simulink model "power_microgrid_v5_battery"  (R2018b)
settings: Solver=ode23tb  StartTime=0.0  StopTime=24*60*60  FixedStep=1/(1000)  MaxStep=60  RelTol=1e-4
PreLoadFcn:
  | load('solar_load_data_24h.mat')
PostLoadFcn:
  | data = xlsread('Domestic_data_all_x3','Sheet1');
  | breakpoints1 = data(2:end,1)'
  | breakpoints2 = data(1,2:end)
  | table_data = data(2:end,2:end)
values from neighbouring files (symbols this model uses):
  SPD_1min = [0 0 0 0 0 0 0 0 0 0 0 0 ... (1441 elements, 1441x1)]    [default_PV_data.mat]
  SPT_1min = [0 60 120 180 240 300 360 420 480 540 600 660 ... (1441 elements, 1441x1)]    [default_PV_data.mat]
libraries: powerlib x155
(part 4 of 5)

== system power_microgrid_v5_battery/House 37 ==
  Clock : Clock
  Complex to Magnitude-Angle : ComplexToMagnitudeAngle  Output=Angle
  Controlled Current Source4 : powerlib/Electrical Sources/Controlled Current Source  Initialize=on  Source_Type=AC  Amplitude=0  Phase=0  Frequency=50  Measurements=None
      settings: SourceProductName=Simscape Electrical
  Gain10 : Gain  Gain=sqrt(2)
  Gain6 : Gain  Gain=-1/230
  Load Data 1-D Lookup Table : Lookup_n-D  NumberOfTableDimensions=1  BreakpointsForDimension1="[0.00\t600.00\t1200.00\t1800.00\t2400.00\t3000.00\t3600.00\t4200.00\t4800.00\t5400.00\t6000.00\t6600.00\t7200.00\t7800.00\t8400.00\t9000.00\t9600.00\t10200.00\t10800.00\t11400.00\t12000.00\t12600.00\t13200.00\t13800.00\t14400.00\t15000.00\t15600.00\t16200.00\t16800.00\t17400.00\t18000.00\t18600.00\t19200.00\t19800.00\t20400.00\t21000.00\t21600.00\t22200.00\t22800.00\t23400.00\t24000.00\t24600.00\t25200.00\t25800.00\t26400.00\t27000.00\t27600.00\t28200.00\t28800.00\t29400.00\t30000.00\t30600.00\t31200.00\t31800.00\t32400.00\t33000.00\t33600.00\t34200.00\t34800.00\t35400.00\t36000.00\t36600.00\t37200.00\t37800.00\t38400.00\t39000.00\t39600.00\t40200.00\t40800.00\t41400.00\t42000.00\t42600.00\t43200.00\t43800.00\t44400.00\t45000.00\t45600.00\t46200.00\t46800.00\t47400.00\t48000.00\t48600.00\t49200.00\t49800.00\t50400.00\t51000.00\t51600.00\t52200.00\t52800.00\t53400.00\t54000.00\t54600.00\t55200.00\t55800.00\t56400.00\t57000.00\t57600.00\t58200.00\t58800.00\t59400.00\t60000.00\t60600.00\t61200.00\t61800.00\t62400.00\t63000.00\t63600.00\t64200.00\t64800.00\t65400.00\t66000.00\t66600.00\t67200.00\t67800.00\t68400.00\t69000.00\t69600.00\t70200.00\t70800.00\t71400.00\t72000.00\t72600.00\t73200.00\t73800.00\t74400.00\t75000.00\t75600.00\t76200.00\t76800.00\t77400.00\t78000.00\t78600.00\t79200.00\t79800.00\t80400.00\t81000.00\t81600.00\t82200.00\t82800.00\t83400.00\t84000.00\t84600.00\t85200.00\t85800.00\t86400.00]"  BeginIndexSearchUsingPreviousIndexResult=on  Table="[287.9\t293.8\t263.0\t241.1\t234.1\t222.8\t214.5\t212.4\t211.1\t207.7\t200.9\t198.4\t194.4\t188.2\t185.8\t183.7\t189.6\t185.1\t179.0\t187.6\t179.7\t177.3\t169.0\t173.0\t169.3\t171.8\t165.9\t166.7\t170.5\t173.6\t179.5\t181.7\t196.2\t192.2\t177.7\t185.2\t250.8\t216.4\t218.6\t232.6\t256.0\t271.2\t292.1\t313.3\t326.6\t375.3\t421.6\t371.9\t375.5\t386.5\t395.4\t389.8\t364.4\t413.6\t395.4\t408.4\t410.4\t379.8\t364.2\t381.0\t383.4\t378.7\t384.3\t387.0\t365.1\t363.6\t369.7\t354.4\t367.8\t353.9\t361.0\t349.4\t377.3\t400.1\t383.7\t374.8\t382.5\t353.8\t359.6\t363.7\t347.9\t331.7\t346.5\t345.9\t334.7\t324.2\t332.7\t349.6\t363.2\t345.4\t350.9\t355.6\t374.0\t393.2\t389.1\t383.8\t404.1\t426.3\t443.7\t449.0\t452.4\t452.9\t477.6\t496.2\t496.4\t518.8\t529.6\t538.5\t545.1\t587.6\t591.8\t593.3\t586.6\t595.1\t603.6\t621.9\t603.6\t607.2\t582.9\t601.9\t605.1\t579.6\t566.2\t557.6\t554.0\t551.3\t552.4\t585.1\t576.4\t564.1\t559.0\t553.1\t536.3\t517.7\t521.5\t519.5\t485.4\t437.7\t418.5\t395.9\t370.8\t353.7\t336.4\t311.0\t287.9]"  InternalRulePriority=Speed  RndMeth=Simplest  InputSameDT=on
  Magnitude-Angle to Complex1 : MagnitudeAngleToComplex
  Snubber3 : powerlib/Elements/Series RLC Branch  LConnTagsString=__new0  RConnTagsString=__new0  BranchType=R  Resistance=1e6  Inductance=1e-3  SetiL0=off  InitialCurrent=0  Capacitance=1e-6  Setx0=off  InitialVoltage=0  Measurements=None
      settings: SourceProductName=Simscape Electrical
  meas cur2 : powerlib/Measurements/Current Measurement  PhasorSimulation=on  OutputType=Complex  PSBequivalent=0
      settings: SourceProductName=Simscape Electrical
  Conn1 : PMIOPort  Side=Left
  Conn2 : PMIOPort  Port=2  Side=Right
  Out1 : Outport
  wires:
  meas cur2/1 -> Out1/1
  Clock/1 -> Load Data 1-D Lookup Table/1
  Magnitude-Angle to Complex1/1 -> Controlled Current Source4/1
  Load Data 1-D Lookup Table/1 -> Gain6/1
  Complex to Magnitude-Angle/1 -> Magnitude-Angle to Complex1/2
  Gain10/1 -> Magnitude-Angle to Complex1/1
  Gain6/1 -> Gain10/1
  [Vsec] -> Complex to Magnitude-Angle/1
  connections:
  Conn1/RConn1 -- meas cur2/LConn1
  Snubber3/LConn1 -- meas cur2/RConn1 -- Controlled Current Source4/RConn1
  Snubber3/RConn1 -- Controlled Current Source4/LConn1 -- Conn2/RConn1

== system power_microgrid_v5_battery/House 38 ==
  Clock : Clock
  Complex to Magnitude-Angle : ComplexToMagnitudeAngle  Output=Angle
  Controlled Current Source4 : powerlib/Electrical Sources/Controlled Current Source  Initialize=on  Source_Type=AC  Amplitude=0  Phase=0  Frequency=50  Measurements=None
      settings: SourceProductName=Simscape Electrical
  Gain10 : Gain  Gain=sqrt(2)
  Gain6 : Gain  Gain=-1/230
  Load Data 1-D Lookup Table : Lookup_n-D  NumberOfTableDimensions=1  BreakpointsForDimension1="[0.00\t600.00\t1200.00\t1800.00\t2400.00\t3000.00\t3600.00\t4200.00\t4800.00\t5400.00\t6000.00\t6600.00\t7200.00\t7800.00\t8400.00\t9000.00\t9600.00\t10200.00\t10800.00\t11400.00\t12000.00\t12600.00\t13200.00\t13800.00\t14400.00\t15000.00\t15600.00\t16200.00\t16800.00\t17400.00\t18000.00\t18600.00\t19200.00\t19800.00\t20400.00\t21000.00\t21600.00\t22200.00\t22800.00\t23400.00\t24000.00\t24600.00\t25200.00\t25800.00\t26400.00\t27000.00\t27600.00\t28200.00\t28800.00\t29400.00\t30000.00\t30600.00\t31200.00\t31800.00\t32400.00\t33000.00\t33600.00\t34200.00\t34800.00\t35400.00\t36000.00\t36600.00\t37200.00\t37800.00\t38400.00\t39000.00\t39600.00\t40200.00\t40800.00\t41400.00\t42000.00\t42600.00\t43200.00\t43800.00\t44400.00\t45000.00\t45600.00\t46200.00\t46800.00\t47400.00\t48000.00\t48600.00\t49200.00\t49800.00\t50400.00\t51000.00\t51600.00\t52200.00\t52800.00\t53400.00\t54000.00\t54600.00\t55200.00\t55800.00\t56400.00\t57000.00\t57600.00\t58200.00\t58800.00\t59400.00\t60000.00\t60600.00\t61200.00\t61800.00\t62400.00\t63000.00\t63600.00\t64200.00\t64800.00\t65400.00\t66000.00\t66600.00\t67200.00\t67800.00\t68400.00\t69000.00\t69600.00\t70200.00\t70800.00\t71400.00\t72000.00\t72600.00\t73200.00\t73800.00\t74400.00\t75000.00\t75600.00\t76200.00\t76800.00\t77400.00\t78000.00\t78600.00\t79200.00\t79800.00\t80400.00\t81000.00\t81600.00\t82200.00\t82800.00\t83400.00\t84000.00\t84600.00\t85200.00\t85800.00\t86400.00]"  BeginIndexSearchUsingPreviousIndexResult=on  Table="[287.9\t293.8\t263.0\t241.1\t234.1\t222.8\t214.5\t212.4\t211.1\t207.7\t200.9\t198.4\t194.4\t188.2\t185.8\t183.7\t189.6\t185.1\t179.0\t187.6\t179.7\t177.3\t169.0\t173.0\t169.3\t171.8\t165.9\t166.7\t170.5\t173.6\t179.5\t181.7\t196.2\t192.2\t177.7\t185.2\t250.8\t216.4\t218.6\t232.6\t256.0\t271.2\t292.1\t313.3\t326.6\t375.3\t421.6\t371.9\t375.5\t386.5\t395.4\t389.8\t364.4\t413.6\t395.4\t408.4\t410.4\t379.8\t364.2\t381.0\t383.4\t378.7\t384.3\t387.0\t365.1\t363.6\t369.7\t354.4\t367.8\t353.9\t361.0\t349.4\t377.3\t400.1\t383.7\t374.8\t382.5\t353.8\t359.6\t363.7\t347.9\t331.7\t346.5\t345.9\t334.7\t324.2\t332.7\t349.6\t363.2\t345.4\t350.9\t355.6\t374.0\t393.2\t389.1\t383.8\t404.1\t426.3\t443.7\t449.0\t452.4\t452.9\t477.6\t496.2\t496.4\t518.8\t529.6\t538.5\t545.1\t587.6\t591.8\t593.3\t586.6\t595.1\t603.6\t621.9\t603.6\t607.2\t582.9\t601.9\t605.1\t579.6\t566.2\t557.6\t554.0\t551.3\t552.4\t585.1\t576.4\t564.1\t559.0\t553.1\t536.3\t517.7\t521.5\t519.5\t485.4\t437.7\t418.5\t395.9\t370.8\t353.7\t336.4\t311.0\t287.9]"  InternalRulePriority=Speed  RndMeth=Simplest  InputSameDT=on
  Magnitude-Angle to Complex1 : MagnitudeAngleToComplex
  Snubber3 : powerlib/Elements/Series RLC Branch  LConnTagsString=__new0  RConnTagsString=__new0  BranchType=R  Resistance=1e6  Inductance=1e-3  SetiL0=off  InitialCurrent=0  Capacitance=1e-6  Setx0=off  InitialVoltage=0  Measurements=None
      settings: SourceProductName=Simscape Electrical
  meas cur2 : powerlib/Measurements/Current Measurement  PhasorSimulation=on  OutputType=Complex  PSBequivalent=0
      settings: SourceProductName=Simscape Electrical
  Conn1 : PMIOPort  Side=Left
  Conn2 : PMIOPort  Port=2  Side=Right
  Out1 : Outport
  wires:
  meas cur2/1 -> Out1/1
  Clock/1 -> Load Data 1-D Lookup Table/1
  Magnitude-Angle to Complex1/1 -> Controlled Current Source4/1
  Load Data 1-D Lookup Table/1 -> Gain6/1
  Complex to Magnitude-Angle/1 -> Magnitude-Angle to Complex1/2
  Gain10/1 -> Magnitude-Angle to Complex1/1
  Gain6/1 -> Gain10/1
  [Vsec] -> Complex to Magnitude-Angle/1
  connections:
  Conn1/RConn1 -- meas cur2/LConn1
  Snubber3/LConn1 -- meas cur2/RConn1 -- Controlled Current Source4/RConn1
  Snubber3/RConn1 -- Controlled Current Source4/LConn1 -- Conn2/RConn1

== system power_microgrid_v5_battery/House 39 ==
  Clock : Clock
  Complex to Magnitude-Angle : ComplexToMagnitudeAngle  Output=Angle
  Controlled Current Source4 : powerlib/Electrical Sources/Controlled Current Source  Initialize=on  Source_Type=AC  Amplitude=0  Phase=0  Frequency=50  Measurements=None
      settings: SourceProductName=Simscape Electrical
  Gain10 : Gain  Gain=sqrt(2)
  Gain6 : Gain  Gain=-1/230
  Load Data 1-D Lookup Table : Lookup_n-D  NumberOfTableDimensions=1  BreakpointsForDimension1="[0.00\t600.00\t1200.00\t1800.00\t2400.00\t3000.00\t3600.00\t4200.00\t4800.00\t5400.00\t6000.00\t6600.00\t7200.00\t7800.00\t8400.00\t9000.00\t9600.00\t10200.00\t10800.00\t11400.00\t12000.00\t12600.00\t13200.00\t13800.00\t14400.00\t15000.00\t15600.00\t16200.00\t16800.00\t17400.00\t18000.00\t18600.00\t19200.00\t19800.00\t20400.00\t21000.00\t21600.00\t22200.00\t22800.00\t23400.00\t24000.00\t24600.00\t25200.00\t25800.00\t26400.00\t27000.00\t27600.00\t28200.00\t28800.00\t29400.00\t30000.00\t30600.00\t31200.00\t31800.00\t32400.00\t33000.00\t33600.00\t34200.00\t34800.00\t35400.00\t36000.00\t36600.00\t37200.00\t37800.00\t38400.00\t39000.00\t39600.00\t40200.00\t40800.00\t41400.00\t42000.00\t42600.00\t43200.00\t43800.00\t44400.00\t45000.00\t45600.00\t46200.00\t46800.00\t47400.00\t48000.00\t48600.00\t49200.00\t49800.00\t50400.00\t51000.00\t51600.00\t52200.00\t52800.00\t53400.00\t54000.00\t54600.00\t55200.00\t55800.00\t56400.00\t57000.00\t57600.00\t58200.00\t58800.00\t59400.00\t60000.00\t60600.00\t61200.00\t61800.00\t62400.00\t63000.00\t63600.00\t64200.00\t64800.00\t65400.00\t66000.00\t66600.00\t67200.00\t67800.00\t68400.00\t69000.00\t69600.00\t70200.00\t70800.00\t71400.00\t72000.00\t72600.00\t73200.00\t73800.00\t74400.00\t75000.00\t75600.00\t76200.00\t76800.00\t77400.00\t78000.00\t78600.00\t79200.00\t79800.00\t80400.00\t81000.00\t81600.00\t82200.00\t82800.00\t83400.00\t84000.00\t84600.00\t85200.00\t85800.00\t86400.00]"  BeginIndexSearchUsingPreviousIndexResult=on  Table="[239.5\t239.3\t230.7\t221.1\t236.7\t224.0\t212.7\t208.1\t198.4\t189.5\t188.5\t190.5\t188.9\t175.4\t181.1\t172.1\t176.3\t181.6\t168.9\t165.2\t160.0\t171.7\t173.3\t158.7\t161.2\t183.5\t182.5\t185.8\t174.7\t172.1\t172.3\t171.8\t196.0\t196.8\t185.5\t191.4\t195.5\t211.1\t225.6\t240.9\t294.0\t327.5\t322.1\t404.9\t489.6\t440.2\t382.2\t398.2\t392.8\t423.0\t511.9\t472.7\t420.5\t405.4\t368.1\t353.8\t392.6\t414.0\t406.8\t409.2\t418.6\t483.6\t444.8\t421.6\t429.0\t444.4\t466.1\t457.6\t477.5\t422.1\t438.5\t445.5\t481.4\t506.4\t471.7\t425.1\t441.5\t411.9\t413.0\t436.9\t429.4\t446.6\t455.6\t465.0\t461.5\t475.0\t453.6\t447.1\t473.5\t480.7\t494.8\t468.2\t491.4\t470.2\t471.6\t525.4\t540.8\t554.3\t565.1\t626.5\t743.4\t744.6\t717.5\t733.8\t778.9\t822.7\t807.8\t820.4\t832.5\t863.5\t825.7\t764.6\t774.5\t717.8\t709.4\t778.0\t738.5\t753.7\t739.0\t770.0\t756.2\t812.2\t746.3\t716.1\t705.9\t737.2\t679.1\t623.3\t583.2\t563.0\t523.2\t504.6\t460.7\t440.9\t392.2\t372.0\t362.3\t339.5\t315.3\t289.8\t274.7\t275.1\t266.0\t264.5\t239.5]"  InternalRulePriority=Speed  RndMeth=Simplest  InputSameDT=on
  Magnitude-Angle to Complex1 : MagnitudeAngleToComplex
  Snubber3 : powerlib/Elements/Series RLC Branch  LConnTagsString=__new0  RConnTagsString=__new0  BranchType=R  Resistance=1e6  Inductance=1e-3  SetiL0=off  InitialCurrent=0  Capacitance=1e-6  Setx0=off  InitialVoltage=0  Measurements=None
      settings: SourceProductName=Simscape Electrical
  meas cur2 : powerlib/Measurements/Current Measurement  PhasorSimulation=on  OutputType=Complex  PSBequivalent=0
      settings: SourceProductName=Simscape Electrical
  Conn1 : PMIOPort  Side=Left
  Conn2 : PMIOPort  Port=2  Side=Right
  Out1 : Outport
  wires:
  Magnitude-Angle to Complex1/1 -> Controlled Current Source4/1
  meas cur2/1 -> Out1/1
  Clock/1 -> Load Data 1-D Lookup Table/1
  Load Data 1-D Lookup Table/1 -> Gain6/1
  [Vsec] -> Complex to Magnitude-Angle/1
  Gain6/1 -> Gain10/1
  Gain10/1 -> Magnitude-Angle to Complex1/1
  Complex to Magnitude-Angle/1 -> Magnitude-Angle to Complex1/2
  connections:
  meas cur2/LConn1 -- Conn1/RConn1
  Snubber3/LConn1 -- Controlled Current Source4/RConn1 -- meas cur2/RConn1
  Snubber3/RConn1 -- Controlled Current Source4/LConn1 -- Conn2/RConn1

== system power_microgrid_v5_battery/House 4 ==
  Clock : Clock
  Complex to Magnitude-Angle : ComplexToMagnitudeAngle  Output=Angle
  Controlled Current Source4 : powerlib/Electrical Sources/Controlled Current Source  Initialize=on  Source_Type=AC  Amplitude=0  Phase=0  Frequency=50  Measurements=None
      settings: SourceProductName=Simscape Electrical
  Gain10 : Gain  Gain=sqrt(2)
  Gain6 : Gain  Gain=-1/230
  Load Data 1-D Lookup Table : Lookup_n-D  NumberOfTableDimensions=1  BreakpointsForDimension1="[0.00\t600.00\t1200.00\t1800.00\t2400.00\t3000.00\t3600.00\t4200.00\t4800.00\t5400.00\t6000.00\t6600.00\t7200.00\t7800.00\t8400.00\t9000.00\t9600.00\t10200.00\t10800.00\t11400.00\t12000.00\t12600.00\t13200.00\t13800.00\t14400.00\t15000.00\t15600.00\t16200.00\t16800.00\t17400.00\t18000.00\t18600.00\t19200.00\t19800.00\t20400.00\t21000.00\t21600.00\t22200.00\t22800.00\t23400.00\t24000.00\t24600.00\t25200.00\t25800.00\t26400.00\t27000.00\t27600.00\t28200.00\t28800.00\t29400.00\t30000.00\t30600.00\t31200.00\t31800.00\t32400.00\t33000.00\t33600.00\t34200.00\t34800.00\t35400.00\t36000.00\t36600.00\t37200.00\t37800.00\t38400.00\t39000.00\t39600.00\t40200.00\t40800.00\t41400.00\t42000.00\t42600.00\t43200.00\t43800.00\t44400.00\t45000.00\t45600.00\t46200.00\t46800.00\t47400.00\t48000.00\t48600.00\t49200.00\t49800.00\t50400.00\t51000.00\t51600.00\t52200.00\t52800.00\t53400.00\t54000.00\t54600.00\t55200.00\t55800.00\t56400.00\t57000.00\t57600.00\t58200.00\t58800.00\t59400.00\t60000.00\t60600.00\t61200.00\t61800.00\t62400.00\t63000.00\t63600.00\t64200.00\t64800.00\t65400.00\t66000.00\t66600.00\t67200.00\t67800.00\t68400.00\t69000.00\t69600.00\t70200.00\t70800.00\t71400.00\t72000.00\t72600.00\t73200.00\t73800.00\t74400.00\t75000.00\t75600.00\t76200.00\t76800.00\t77400.00\t78000.00\t78600.00\t79200.00\t79800.00\t80400.00\t81000.00\t81600.00\t82200.00\t82800.00\t83400.00\t84000.00\t84600.00\t85200.00\t85800.00\t86400.00]"  BeginIndexSearchUsingPreviousIndexResult=on  Table="[179.5\t163.3\t152.9\t132.5\t118.9\t111.3\t124.6\t103.3\t83.5\t81.2\t85.9\t85.2\t91.9\t95.6\t95.9\t81.8\t83.7\t86.7\t93.8\t81.2\t92.7\t99.4\t112.6\t88.2\t85.6\t78.4\t88.4\t93.9\t86.1\t86.0\t111.7\t143.5\t122.7\t136.8\t142.2\t135.1\t145.6\t141.8\t152.1\t140.3\t167.9\t256.6\t226.1\t263.8\t283.9\t303.3\t279.5\t294.9\t282.3\t288.8\t333.5\t360.9\t421.4\t494.2\t392.5\t439.7\t395.9\t394.4\t364.9\t353.0\t359.1\t370.9\t398.5\t447.4\t344.5\t330.8\t306.8\t331.3\t331.9\t307.6\t371.3\t387.4\t376.6\t360.2\t414.1\t445.1\t411.1\t389.5\t425.2\t340.0\t316.3\t332.8\t352.3\t301.8\t261.8\t298.1\t350.9\t327.8\t296.5\t319.6\t368.4\t327.2\t265.7\t277.9\t292.9\t301.4\t377.9\t336.0\t324.6\t353.8\t389.7\t355.9\t328.4\t325.9\t378.1\t338.0\t379.1\t414.8\t418.1\t464.8\t488.1\t489.1\t485.7\t581.3\t579.7\t526.2\t551.4\t618.6\t628.5\t578.8\t553.3\t481.5\t455.6\t487.9\t507.3\t497.6\t515.4\t510.2\t490.5\t500.5\t494.1\t532.9\t506.5\t466.6\t438.0\t385.4\t381.2\t385.9\t351.7\t371.3\t340.8\t320.2\t277.0\t228.9\t179.5]"  InternalRulePriority=Speed  RndMeth=Simplest  InputSameDT=on
  Magnitude-Angle to Complex1 : MagnitudeAngleToComplex
  Snubber3 : powerlib/Elements/Series RLC Branch  LConnTagsString=__new0  RConnTagsString=__new0  BranchType=R  Resistance=1e6  Inductance=1e-3  SetiL0=off  InitialCurrent=0  Capacitance=1e-6  Setx0=off  InitialVoltage=0  Measurements=None
      settings: SourceProductName=Simscape Electrical
  meas cur2 : powerlib/Measurements/Current Measurement  PhasorSimulation=on  OutputType=Complex  PSBequivalent=0
      settings: SourceProductName=Simscape Electrical
  Conn1 : PMIOPort  Side=Left
  Conn2 : PMIOPort  Port=2  Side=Right
  Out1 : Outport
  wires:
  meas cur2/1 -> Out1/1
  Clock/1 -> Load Data 1-D Lookup Table/1
  Magnitude-Angle to Complex1/1 -> Controlled Current Source4/1
  Load Data 1-D Lookup Table/1 -> Gain6/1
  Complex to Magnitude-Angle/1 -> Magnitude-Angle to Complex1/2
  Gain10/1 -> Magnitude-Angle to Complex1/1
  Gain6/1 -> Gain10/1
  [Vsec] -> Complex to Magnitude-Angle/1
  connections:
  Conn1/RConn1 -- meas cur2/LConn1
  Snubber3/LConn1 -- meas cur2/RConn1 -- Controlled Current Source4/RConn1
  Snubber3/RConn1 -- Controlled Current Source4/LConn1 -- Conn2/RConn1

== system power_microgrid_v5_battery/House 40 ==
  Clock : Clock
  Complex to Magnitude-Angle : ComplexToMagnitudeAngle  Output=Angle
  Controlled Current Source4 : powerlib/Electrical Sources/Controlled Current Source  Initialize=on  Source_Type=AC  Amplitude=0  Phase=0  Frequency=50  Measurements=None
      settings: SourceProductName=Simscape Electrical
  Gain10 : Gain  Gain=sqrt(2)
  Gain6 : Gain  Gain=-1/230
  Load Data 1-D Lookup Table : Lookup_n-D  NumberOfTableDimensions=1  BreakpointsForDimension1="[0.00\t600.00\t1200.00\t1800.00\t2400.00\t3000.00\t3600.00\t4200.00\t4800.00\t5400.00\t6000.00\t6600.00\t7200.00\t7800.00\t8400.00\t9000.00\t9600.00\t10200.00\t10800.00\t11400.00\t12000.00\t12600.00\t13200.00\t13800.00\t14400.00\t15000.00\t15600.00\t16200.00\t16800.00\t17400.00\t18000.00\t18600.00\t19200.00\t19800.00\t20400.00\t21000.00\t21600.00\t22200.00\t22800.00\t23400.00\t24000.00\t24600.00\t25200.00\t25800.00\t26400.00\t27000.00\t27600.00\t28200.00\t28800.00\t29400.00\t30000.00\t30600.00\t31200.00\t31800.00\t32400.00\t33000.00\t33600.00\t34200.00\t34800.00\t35400.00\t36000.00\t36600.00\t37200.00\t37800.00\t38400.00\t39000.00\t39600.00\t40200.00\t40800.00\t41400.00\t42000.00\t42600.00\t43200.00\t43800.00\t44400.00\t45000.00\t45600.00\t46200.00\t46800.00\t47400.00\t48000.00\t48600.00\t49200.00\t49800.00\t50400.00\t51000.00\t51600.00\t52200.00\t52800.00\t53400.00\t54000.00\t54600.00\t55200.00\t55800.00\t56400.00\t57000.00\t57600.00\t58200.00\t58800.00\t59400.00\t60000.00\t60600.00\t61200.00\t61800.00\t62400.00\t63000.00\t63600.00\t64200.00\t64800.00\t65400.00\t66000.00\t66600.00\t67200.00\t67800.00\t68400.00\t69000.00\t69600.00\t70200.00\t70800.00\t71400.00\t72000.00\t72600.00\t73200.00\t73800.00\t74400.00\t75000.00\t75600.00\t76200.00\t76800.00\t77400.00\t78000.00\t78600.00\t79200.00\t79800.00\t80400.00\t81000.00\t81600.00\t82200.00\t82800.00\t83400.00\t84000.00\t84600.00\t85200.00\t85800.00\t86400.00]"  BeginIndexSearchUsingPreviousIndexResult=on  Table="[239.5\t239.3\t230.7\t221.1\t236.7\t224.0\t212.7\t208.1\t198.4\t189.5\t188.5\t190.5\t188.9\t175.4\t181.1\t172.1\t176.3\t181.6\t168.9\t165.2\t160.0\t171.7\t173.3\t158.7\t161.2\t183.5\t182.5\t185.8\t174.7\t172.1\t172.3\t171.8\t196.0\t196.8\t185.5\t191.4\t195.5\t211.1\t225.6\t240.9\t294.0\t327.5\t322.1\t404.9\t489.6\t440.2\t382.2\t398.2\t392.8\t423.0\t511.9\t472.7\t420.5\t405.4\t368.1\t353.8\t392.6\t414.0\t406.8\t409.2\t418.6\t483.6\t444.8\t421.6\t429.0\t444.4\t466.1\t457.6\t477.5\t422.1\t438.5\t445.5\t481.4\t506.4\t471.7\t425.1\t441.5\t411.9\t413.0\t436.9\t429.4\t446.6\t455.6\t465.0\t461.5\t475.0\t453.6\t447.1\t473.5\t480.7\t494.8\t468.2\t491.4\t470.2\t471.6\t525.4\t540.8\t554.3\t565.1\t626.5\t743.4\t744.6\t717.5\t733.8\t778.9\t822.7\t807.8\t820.4\t832.5\t863.5\t825.7\t764.6\t774.5\t717.8\t709.4\t778.0\t738.5\t753.7\t739.0\t770.0\t756.2\t812.2\t746.3\t716.1\t705.9\t737.2\t679.1\t623.3\t583.2\t563.0\t523.2\t504.6\t460.7\t440.9\t392.2\t372.0\t362.3\t339.5\t315.3\t289.8\t274.7\t275.1\t266.0\t264.5\t239.5]"  InternalRulePriority=Speed  RndMeth=Simplest  InputSameDT=on
  Magnitude-Angle to Complex1 : MagnitudeAngleToComplex
  Snubber3 : powerlib/Elements/Series RLC Branch  LConnTagsString=__new0  RConnTagsString=__new0  BranchType=R  Resistance=1e6  Inductance=1e-3  SetiL0=off  InitialCurrent=0  Capacitance=1e-6  Setx0=off  InitialVoltage=0  Measurements=None
      settings: SourceProductName=Simscape Electrical
  meas cur2 : powerlib/Measurements/Current Measurement  PhasorSimulation=on  OutputType=Complex  PSBequivalent=0
      settings: SourceProductName=Simscape Electrical
  Conn1 : PMIOPort  Side=Left
  Conn2 : PMIOPort  Port=2  Side=Right
  Out1 : Outport
  wires:
  meas cur2/1 -> Out1/1
  Clock/1 -> Load Data 1-D Lookup Table/1
  Magnitude-Angle to Complex1/1 -> Controlled Current Source4/1
  Load Data 1-D Lookup Table/1 -> Gain6/1
  Complex to Magnitude-Angle/1 -> Magnitude-Angle to Complex1/2
  Gain10/1 -> Magnitude-Angle to Complex1/1
  Gain6/1 -> Gain10/1
  [Vsec] -> Complex to Magnitude-Angle/1
  connections:
  Controlled Current Source4/LConn1 -- Conn2/RConn1 -- Snubber3/RConn1
  Controlled Current Source4/RConn1 -- meas cur2/RConn1 -- Snubber3/LConn1
  Conn1/RConn1 -- meas cur2/LConn1

== system power_microgrid_v5_battery/House 41 ==
  Clock : Clock
  Complex to Magnitude-Angle : ComplexToMagnitudeAngle  Output=Angle
  Controlled Current Source4 : powerlib/Electrical Sources/Controlled Current Source  Initialize=on  Source_Type=AC  Amplitude=0  Phase=0  Frequency=50  Measurements=None
      settings: SourceProductName=Simscape Electrical
  Gain10 : Gain  Gain=sqrt(2)
  Gain6 : Gain  Gain=-1/230
  Load Data 1-D Lookup Table : Lookup_n-D  NumberOfTableDimensions=1  BreakpointsForDimension1="[0.00\t600.00\t1200.00\t1800.00\t2400.00\t3000.00\t3600.00\t4200.00\t4800.00\t5400.00\t6000.00\t6600.00\t7200.00\t7800.00\t8400.00\t9000.00\t9600.00\t10200.00\t10800.00\t11400.00\t12000.00\t12600.00\t13200.00\t13800.00\t14400.00\t15000.00\t15600.00\t16200.00\t16800.00\t17400.00\t18000.00\t18600.00\t19200.00\t19800.00\t20400.00\t21000.00\t21600.00\t22200.00\t22800.00\t23400.00\t24000.00\t24600.00\t25200.00\t25800.00\t26400.00\t27000.00\t27600.00\t28200.00\t28800.00\t29400.00\t30000.00\t30600.00\t31200.00\t31800.00\t32400.00\t33000.00\t33600.00\t34200.00\t34800.00\t35400.00\t36000.00\t36600.00\t37200.00\t37800.00\t38400.00\t39000.00\t39600.00\t40200.00\t40800.00\t41400.00\t42000.00\t42600.00\t43200.00\t43800.00\t44400.00\t45000.00\t45600.00\t46200.00\t46800.00\t47400.00\t48000.00\t48600.00\t49200.00\t49800.00\t50400.00\t51000.00\t51600.00\t52200.00\t52800.00\t53400.00\t54000.00\t54600.00\t55200.00\t55800.00\t56400.00\t57000.00\t57600.00\t58200.00\t58800.00\t59400.00\t60000.00\t60600.00\t61200.00\t61800.00\t62400.00\t63000.00\t63600.00\t64200.00\t64800.00\t65400.00\t66000.00\t66600.00\t67200.00\t67800.00\t68400.00\t69000.00\t69600.00\t70200.00\t70800.00\t71400.00\t72000.00\t72600.00\t73200.00\t73800.00\t74400.00\t75000.00\t75600.00\t76200.00\t76800.00\t77400.00\t78000.00\t78600.00\t79200.00\t79800.00\t80400.00\t81000.00\t81600.00\t82200.00\t82800.00\t83400.00\t84000.00\t84600.00\t85200.00\t85800.00\t86400.00]"  BeginIndexSearchUsingPreviousIndexResult=on  Table="[179.5\t163.3\t152.9\t132.5\t118.9\t111.3\t124.6\t103.3\t83.5\t81.2\t85.9\t85.2\t91.9\t95.6\t95.9\t81.8\t83.7\t86.7\t93.8\t81.2\t92.7\t99.4\t112.6\t88.2\t85.6\t78.4\t88.4\t93.9\t86.1\t86.0\t111.7\t143.5\t122.7\t136.8\t142.2\t135.1\t145.6\t141.8\t152.1\t140.3\t167.9\t256.6\t226.1\t263.8\t283.9\t303.3\t279.5\t294.9\t282.3\t288.8\t333.5\t360.9\t421.4\t494.2\t392.5\t439.7\t395.9\t394.4\t364.9\t353.0\t359.1\t370.9\t398.5\t447.4\t344.5\t330.8\t306.8\t331.3\t331.9\t307.6\t371.3\t387.4\t376.6\t360.2\t414.1\t445.1\t411.1\t389.5\t425.2\t340.0\t316.3\t332.8\t352.3\t301.8\t261.8\t298.1\t350.9\t327.8\t296.5\t319.6\t368.4\t327.2\t265.7\t277.9\t292.9\t301.4\t377.9\t336.0\t324.6\t353.8\t389.7\t355.9\t328.4\t325.9\t378.1\t338.0\t379.1\t414.8\t418.1\t464.8\t488.1\t489.1\t485.7\t581.3\t579.7\t526.2\t551.4\t618.6\t628.5\t578.8\t553.3\t481.5\t455.6\t487.9\t507.3\t497.6\t515.4\t510.2\t490.5\t500.5\t494.1\t532.9\t506.5\t466.6\t438.0\t385.4\t381.2\t385.9\t351.7\t371.3\t340.8\t320.2\t277.0\t228.9\t179.5]"  InternalRulePriority=Speed  RndMeth=Simplest  InputSameDT=on
  Magnitude-Angle to Complex1 : MagnitudeAngleToComplex
  Snubber3 : powerlib/Elements/Series RLC Branch  LConnTagsString=__new0  RConnTagsString=__new0  BranchType=R  Resistance=1e6  Inductance=1e-3  SetiL0=off  InitialCurrent=0  Capacitance=1e-6  Setx0=off  InitialVoltage=0  Measurements=None
      settings: SourceProductName=Simscape Electrical
  meas cur2 : powerlib/Measurements/Current Measurement  PhasorSimulation=on  OutputType=Complex  PSBequivalent=0
      settings: SourceProductName=Simscape Electrical
  Conn1 : PMIOPort  Side=Left
  Conn2 : PMIOPort  Port=2  Side=Right
  Out1 : Outport
  wires:
  meas cur2/1 -> Out1/1
  Clock/1 -> Load Data 1-D Lookup Table/1
  Magnitude-Angle to Complex1/1 -> Controlled Current Source4/1
  Load Data 1-D Lookup Table/1 -> Gain6/1
  Complex to Magnitude-Angle/1 -> Magnitude-Angle to Complex1/2
  Gain10/1 -> Magnitude-Angle to Complex1/1
  Gain6/1 -> Gain10/1
  [Vsec] -> Complex to Magnitude-Angle/1
  connections:
  Conn1/RConn1 -- meas cur2/LConn1
  Snubber3/LConn1 -- meas cur2/RConn1 -- Controlled Current Source4/RConn1
  Snubber3/RConn1 -- Controlled Current Source4/LConn1 -- Conn2/RConn1

== system power_microgrid_v5_battery/House 5 ==
  Clock : Clock
  Complex to Magnitude-Angle : ComplexToMagnitudeAngle  Output=Angle
  Controlled Current Source4 : powerlib/Electrical Sources/Controlled Current Source  Initialize=on  Source_Type=AC  Amplitude=0  Phase=0  Frequency=50  Measurements=None
      settings: SourceProductName=Simscape Electrical
  Gain10 : Gain  Gain=sqrt(2)
  Gain6 : Gain  Gain=-1/230
  Load Data 1-D Lookup Table : Lookup_n-D  NumberOfTableDimensions=1  BreakpointsForDimension1="[0.00\t600.00\t1200.00\t1800.00\t2400.00\t3000.00\t3600.00\t4200.00\t4800.00\t5400.00\t6000.00\t6600.00\t7200.00\t7800.00\t8400.00\t9000.00\t9600.00\t10200.00\t10800.00\t11400.00\t12000.00\t12600.00\t13200.00\t13800.00\t14400.00\t15000.00\t15600.00\t16200.00\t16800.00\t17400.00\t18000.00\t18600.00\t19200.00\t19800.00\t20400.00\t21000.00\t21600.00\t22200.00\t22800.00\t23400.00\t24000.00\t24600.00\t25200.00\t25800.00\t26400.00\t27000.00\t27600.00\t28200.00\t28800.00\t29400.00\t30000.00\t30600.00\t31200.00\t31800.00\t32400.00\t33000.00\t33600.00\t34200.00\t34800.00\t35400.00\t36000.00\t36600.00\t37200.00\t37800.00\t38400.00\t39000.00\t39600.00\t40200.00\t40800.00\t41400.00\t42000.00\t42600.00\t43200.00\t43800.00\t44400.00\t45000.00\t45600.00\t46200.00\t46800.00\t47400.00\t48000.00\t48600.00\t49200.00\t49800.00\t50400.00\t51000.00\t51600.00\t52200.00\t52800.00\t53400.00\t54000.00\t54600.00\t55200.00\t55800.00\t56400.00\t57000.00\t57600.00\t58200.00\t58800.00\t59400.00\t60000.00\t60600.00\t61200.00\t61800.00\t62400.00\t63000.00\t63600.00\t64200.00\t64800.00\t65400.00\t66000.00\t66600.00\t67200.00\t67800.00\t68400.00\t69000.00\t69600.00\t70200.00\t70800.00\t71400.00\t72000.00\t72600.00\t73200.00\t73800.00\t74400.00\t75000.00\t75600.00\t76200.00\t76800.00\t77400.00\t78000.00\t78600.00\t79200.00\t79800.00\t80400.00\t81000.00\t81600.00\t82200.00\t82800.00\t83400.00\t84000.00\t84600.00\t85200.00\t85800.00\t86400.00]"  BeginIndexSearchUsingPreviousIndexResult=on  Table="[179.5\t163.3\t152.9\t132.5\t118.9\t111.3\t124.6\t103.3\t83.5\t81.2\t85.9\t85.2\t91.9\t95.6\t95.9\t81.8\t83.7\t86.7\t93.8\t81.2\t92.7\t99.4\t112.6\t88.2\t85.6\t78.4\t88.4\t93.9\t86.1\t86.0\t111.7\t143.5\t122.7\t136.8\t142.2\t135.1\t145.6\t141.8\t152.1\t140.3\t167.9\t256.6\t226.1\t263.8\t283.9\t303.3\t279.5\t294.9\t282.3\t288.8\t333.5\t360.9\t421.4\t494.2\t392.5\t439.7\t395.9\t394.4\t364.9\t353.0\t359.1\t370.9\t398.5\t447.4\t344.5\t330.8\t306.8\t331.3\t331.9\t307.6\t371.3\t387.4\t376.6\t360.2\t414.1\t445.1\t411.1\t389.5\t425.2\t340.0\t316.3\t332.8\t352.3\t301.8\t261.8\t298.1\t350.9\t327.8\t296.5\t319.6\t368.4\t327.2\t265.7\t277.9\t292.9\t301.4\t377.9\t336.0\t324.6\t353.8\t389.7\t355.9\t328.4\t325.9\t378.1\t338.0\t379.1\t414.8\t418.1\t464.8\t488.1\t489.1\t485.7\t581.3\t579.7\t526.2\t551.4\t618.6\t628.5\t578.8\t553.3\t481.5\t455.6\t487.9\t507.3\t497.6\t515.4\t510.2\t490.5\t500.5\t494.1\t532.9\t506.5\t466.6\t438.0\t385.4\t381.2\t385.9\t351.7\t371.3\t340.8\t320.2\t277.0\t228.9\t179.5]"  InternalRulePriority=Speed  RndMeth=Simplest  InputSameDT=on
  Magnitude-Angle to Complex1 : MagnitudeAngleToComplex
  Snubber3 : powerlib/Elements/Series RLC Branch  LConnTagsString=__new0  RConnTagsString=__new0  BranchType=R  Resistance=1e6  Inductance=1e-3  SetiL0=off  InitialCurrent=0  Capacitance=1e-6  Setx0=off  InitialVoltage=0  Measurements=None
      settings: SourceProductName=Simscape Electrical
  meas cur2 : powerlib/Measurements/Current Measurement  PhasorSimulation=on  OutputType=Complex  PSBequivalent=0
      settings: SourceProductName=Simscape Electrical
  Conn1 : PMIOPort  Side=Left
  Conn2 : PMIOPort  Port=2  Side=Right
  Out1 : Outport
  wires:
  meas cur2/1 -> Out1/1
  Clock/1 -> Load Data 1-D Lookup Table/1
  Magnitude-Angle to Complex1/1 -> Controlled Current Source4/1
  Load Data 1-D Lookup Table/1 -> Gain6/1
  Complex to Magnitude-Angle/1 -> Magnitude-Angle to Complex1/2
  Gain10/1 -> Magnitude-Angle to Complex1/1
  Gain6/1 -> Gain10/1
  [Vsec] -> Complex to Magnitude-Angle/1
  connections:
  Conn1/RConn1 -- meas cur2/LConn1
  Snubber3/LConn1 -- meas cur2/RConn1 -- Controlled Current Source4/RConn1
  Snubber3/RConn1 -- Controlled Current Source4/LConn1 -- Conn2/RConn1

== system power_microgrid_v5_battery/House 6 ==
  Clock : Clock
  Complex to Magnitude-Angle : ComplexToMagnitudeAngle  Output=Angle
  Controlled Current Source4 : powerlib/Electrical Sources/Controlled Current Source  Initialize=on  Source_Type=AC  Amplitude=0  Phase=0  Frequency=50  Measurements=None
      settings: SourceProductName=Simscape Electrical
  Gain10 : Gain  Gain=sqrt(2)
  Gain6 : Gain  Gain=-1/230
  Load Data 1-D Lookup Table : Lookup_n-D  NumberOfTableDimensions=1  BreakpointsForDimension1="[0.00\t600.00\t1200.00\t1800.00\t2400.00\t3000.00\t3600.00\t4200.00\t4800.00\t5400.00\t6000.00\t6600.00\t7200.00\t7800.00\t8400.00\t9000.00\t9600.00\t10200.00\t10800.00\t11400.00\t12000.00\t12600.00\t13200.00\t13800.00\t14400.00\t15000.00\t15600.00\t16200.00\t16800.00\t17400.00\t18000.00\t18600.00\t19200.00\t19800.00\t20400.00\t21000.00\t21600.00\t22200.00\t22800.00\t23400.00\t24000.00\t24600.00\t25200.00\t25800.00\t26400.00\t27000.00\t27600.00\t28200.00\t28800.00\t29400.00\t30000.00\t30600.00\t31200.00\t31800.00\t32400.00\t33000.00\t33600.00\t34200.00\t34800.00\t35400.00\t36000.00\t36600.00\t37200.00\t37800.00\t38400.00\t39000.00\t39600.00\t40200.00\t40800.00\t41400.00\t42000.00\t42600.00\t43200.00\t43800.00\t44400.00\t45000.00\t45600.00\t46200.00\t46800.00\t47400.00\t48000.00\t48600.00\t49200.00\t49800.00\t50400.00\t51000.00\t51600.00\t52200.00\t52800.00\t53400.00\t54000.00\t54600.00\t55200.00\t55800.00\t56400.00\t57000.00\t57600.00\t58200.00\t58800.00\t59400.00\t60000.00\t60600.00\t61200.00\t61800.00\t62400.00\t63000.00\t63600.00\t64200.00\t64800.00\t65400.00\t66000.00\t66600.00\t67200.00\t67800.00\t68400.00\t69000.00\t69600.00\t70200.00\t70800.00\t71400.00\t72000.00\t72600.00\t73200.00\t73800.00\t74400.00\t75000.00\t75600.00\t76200.00\t76800.00\t77400.00\t78000.00\t78600.00\t79200.00\t79800.00\t80400.00\t81000.00\t81600.00\t82200.00\t82800.00\t83400.00\t84000.00\t84600.00\t85200.00\t85800.00\t86400.00]"  BeginIndexSearchUsingPreviousIndexResult=on  Table="[179.5\t163.3\t152.9\t132.5\t118.9\t111.3\t124.6\t103.3\t83.5\t81.2\t85.9\t85.2\t91.9\t95.6\t95.9\t81.8\t83.7\t86.7\t93.8\t81.2\t92.7\t99.4\t112.6\t88.2\t85.6\t78.4\t88.4\t93.9\t86.1\t86.0\t111.7\t143.5\t122.7\t136.8\t142.2\t135.1\t145.6\t141.8\t152.1\t140.3\t167.9\t256.6\t226.1\t263.8\t283.9\t303.3\t279.5\t294.9\t282.3\t288.8\t333.5\t360.9\t421.4\t494.2\t392.5\t439.7\t395.9\t394.4\t364.9\t353.0\t359.1\t370.9\t398.5\t447.4\t344.5\t330.8\t306.8\t331.3\t331.9\t307.6\t371.3\t387.4\t376.6\t360.2\t414.1\t445.1\t411.1\t389.5\t425.2\t340.0\t316.3\t332.8\t352.3\t301.8\t261.8\t298.1\t350.9\t327.8\t296.5\t319.6\t368.4\t327.2\t265.7\t277.9\t292.9\t301.4\t377.9\t336.0\t324.6\t353.8\t389.7\t355.9\t328.4\t325.9\t378.1\t338.0\t379.1\t414.8\t418.1\t464.8\t488.1\t489.1\t485.7\t581.3\t579.7\t526.2\t551.4\t618.6\t628.5\t578.8\t553.3\t481.5\t455.6\t487.9\t507.3\t497.6\t515.4\t510.2\t490.5\t500.5\t494.1\t532.9\t506.5\t466.6\t438.0\t385.4\t381.2\t385.9\t351.7\t371.3\t340.8\t320.2\t277.0\t228.9\t179.5]"  InternalRulePriority=Speed  RndMeth=Simplest  InputSameDT=on
  Magnitude-Angle to Complex1 : MagnitudeAngleToComplex
  Snubber3 : powerlib/Elements/Series RLC Branch  LConnTagsString=__new0  RConnTagsString=__new0  BranchType=R  Resistance=1e6  Inductance=1e-3  SetiL0=off  InitialCurrent=0  Capacitance=1e-6  Setx0=off  InitialVoltage=0  Measurements=None
      settings: SourceProductName=Simscape Electrical
  meas cur2 : powerlib/Measurements/Current Measurement  PhasorSimulation=on  OutputType=Complex  PSBequivalent=0
      settings: SourceProductName=Simscape Electrical
  Conn1 : PMIOPort  Side=Left
  Conn2 : PMIOPort  Port=2  Side=Right
  Out1 : Outport
  wires:
  meas cur2/1 -> Out1/1
  Clock/1 -> Load Data 1-D Lookup Table/1
  Magnitude-Angle to Complex1/1 -> Controlled Current Source4/1
  Load Data 1-D Lookup Table/1 -> Gain6/1
  Complex to Magnitude-Angle/1 -> Magnitude-Angle to Complex1/2
  Gain10/1 -> Magnitude-Angle to Complex1/1
  Gain6/1 -> Gain10/1
  [Vsec] -> Complex to Magnitude-Angle/1
  connections:
  Conn1/RConn1 -- meas cur2/LConn1
  Snubber3/LConn1 -- meas cur2/RConn1 -- Controlled Current Source4/RConn1
  Snubber3/RConn1 -- Controlled Current Source4/LConn1 -- Conn2/RConn1

== system power_microgrid_v5_battery/House 7 ==
  Clock : Clock
  Complex to Magnitude-Angle : ComplexToMagnitudeAngle  Output=Angle
  Controlled Current Source4 : powerlib/Electrical Sources/Controlled Current Source  Initialize=on  Source_Type=AC  Amplitude=0  Phase=0  Frequency=50  Measurements=None
      settings: SourceProductName=Simscape Electrical
  Gain10 : Gain  Gain=sqrt(2)
  Gain6 : Gain  Gain=-1/230
  Load Data 1-D Lookup Table : Lookup_n-D  NumberOfTableDimensions=1  BreakpointsForDimension1="[0.00\t600.00\t1200.00\t1800.00\t2400.00\t3000.00\t3600.00\t4200.00\t4800.00\t5400.00\t6000.00\t6600.00\t7200.00\t7800.00\t8400.00\t9000.00\t9600.00\t10200.00\t10800.00\t11400.00\t12000.00\t12600.00\t13200.00\t13800.00\t14400.00\t15000.00\t15600.00\t16200.00\t16800.00\t17400.00\t18000.00\t18600.00\t19200.00\t19800.00\t20400.00\t21000.00\t21600.00\t22200.00\t22800.00\t23400.00\t24000.00\t24600.00\t25200.00\t25800.00\t26400.00\t27000.00\t27600.00\t28200.00\t28800.00\t29400.00\t30000.00\t30600.00\t31200.00\t31800.00\t32400.00\t33000.00\t33600.00\t34200.00\t34800.00\t35400.00\t36000.00\t36600.00\t37200.00\t37800.00\t38400.00\t39000.00\t39600.00\t40200.00\t40800.00\t41400.00\t42000.00\t42600.00\t43200.00\t43800.00\t44400.00\t45000.00\t45600.00\t46200.00\t46800.00\t47400.00\t48000.00\t48600.00\t49200.00\t49800.00\t50400.00\t51000.00\t51600.00\t52200.00\t52800.00\t53400.00\t54000.00\t54600.00\t55200.00\t55800.00\t56400.00\t57000.00\t57600.00\t58200.00\t58800.00\t59400.00\t60000.00\t60600.00\t61200.00\t61800.00\t62400.00\t63000.00\t63600.00\t64200.00\t64800.00\t65400.00\t66000.00\t66600.00\t67200.00\t67800.00\t68400.00\t69000.00\t69600.00\t70200.00\t70800.00\t71400.00\t72000.00\t72600.00\t73200.00\t73800.00\t74400.00\t75000.00\t75600.00\t76200.00\t76800.00\t77400.00\t78000.00\t78600.00\t79200.00\t79800.00\t80400.00\t81000.00\t81600.00\t82200.00\t82800.00\t83400.00\t84000.00\t84600.00\t85200.00\t85800.00\t86400.00]"  BeginIndexSearchUsingPreviousIndexResult=on  Table="[179.5\t163.3\t152.9\t132.5\t118.9\t111.3\t124.6\t103.3\t83.5\t81.2\t85.9\t85.2\t91.9\t95.6\t95.9\t81.8\t83.7\t86.7\t93.8\t81.2\t92.7\t99.4\t112.6\t88.2\t85.6\t78.4\t88.4\t93.9\t86.1\t86.0\t111.7\t143.5\t122.7\t136.8\t142.2\t135.1\t145.6\t141.8\t152.1\t140.3\t167.9\t256.6\t226.1\t263.8\t283.9\t303.3\t279.5\t294.9\t282.3\t288.8\t333.5\t360.9\t421.4\t494.2\t392.5\t439.7\t395.9\t394.4\t364.9\t353.0\t359.1\t370.9\t398.5\t447.4\t344.5\t330.8\t306.8\t331.3\t331.9\t307.6\t371.3\t387.4\t376.6\t360.2\t414.1\t445.1\t411.1\t389.5\t425.2\t340.0\t316.3\t332.8\t352.3\t301.8\t261.8\t298.1\t350.9\t327.8\t296.5\t319.6\t368.4\t327.2\t265.7\t277.9\t292.9\t301.4\t377.9\t336.0\t324.6\t353.8\t389.7\t355.9\t328.4\t325.9\t378.1\t338.0\t379.1\t414.8\t418.1\t464.8\t488.1\t489.1\t485.7\t581.3\t579.7\t526.2\t551.4\t618.6\t628.5\t578.8\t553.3\t481.5\t455.6\t487.9\t507.3\t497.6\t515.4\t510.2\t490.5\t500.5\t494.1\t532.9\t506.5\t466.6\t438.0\t385.4\t381.2\t385.9\t351.7\t371.3\t340.8\t320.2\t277.0\t228.9\t179.5]"  InternalRulePriority=Speed  RndMeth=Simplest  InputSameDT=on
  Magnitude-Angle to Complex1 : MagnitudeAngleToComplex
  Snubber3 : powerlib/Elements/Series RLC Branch  LConnTagsString=__new0  RConnTagsString=__new0  BranchType=R  Resistance=1e6  Inductance=1e-3  SetiL0=off  InitialCurrent=0  Capacitance=1e-6  Setx0=off  InitialVoltage=0  Measurements=None
      settings: SourceProductName=Simscape Electrical
  meas cur2 : powerlib/Measurements/Current Measurement  PhasorSimulation=on  OutputType=Complex  PSBequivalent=0
      settings: SourceProductName=Simscape Electrical
  Conn1 : PMIOPort  Side=Left
  Conn2 : PMIOPort  Port=2  Side=Right
  Out1 : Outport
  wires:
  meas cur2/1 -> Out1/1
  Clock/1 -> Load Data 1-D Lookup Table/1
  Magnitude-Angle to Complex1/1 -> Controlled Current Source4/1
  Load Data 1-D Lookup Table/1 -> Gain6/1
  Complex to Magnitude-Angle/1 -> Magnitude-Angle to Complex1/2
  Gain10/1 -> Magnitude-Angle to Complex1/1
  Gain6/1 -> Gain10/1
  [Vsec] -> Complex to Magnitude-Angle/1
  connections:
  Conn1/RConn1 -- meas cur2/LConn1
  Snubber3/LConn1 -- meas cur2/RConn1 -- Controlled Current Source4/RConn1
  Snubber3/RConn1 -- Controlled Current Source4/LConn1 -- Conn2/RConn1

== system power_microgrid_v5_battery/House 8 ==
  Clock : Clock
  Complex to Magnitude-Angle : ComplexToMagnitudeAngle  Output=Angle
  Controlled Current Source4 : powerlib/Electrical Sources/Controlled Current Source  Initialize=on  Source_Type=AC  Amplitude=0  Phase=0  Frequency=50  Measurements=None
      settings: SourceProductName=Simscape Electrical
  Gain10 : Gain  Gain=sqrt(2)
  Gain6 : Gain  Gain=-1/230
  Load Data 1-D Lookup Table : Lookup_n-D  NumberOfTableDimensions=1  BreakpointsForDimension1="[0.00\t600.00\t1200.00\t1800.00\t2400.00\t3000.00\t3600.00\t4200.00\t4800.00\t5400.00\t6000.00\t6600.00\t7200.00\t7800.00\t8400.00\t9000.00\t9600.00\t10200.00\t10800.00\t11400.00\t12000.00\t12600.00\t13200.00\t13800.00\t14400.00\t15000.00\t15600.00\t16200.00\t16800.00\t17400.00\t18000.00\t18600.00\t19200.00\t19800.00\t20400.00\t21000.00\t21600.00\t22200.00\t22800.00\t23400.00\t24000.00\t24600.00\t25200.00\t25800.00\t26400.00\t27000.00\t27600.00\t28200.00\t28800.00\t29400.00\t30000.00\t30600.00\t31200.00\t31800.00\t32400.00\t33000.00\t33600.00\t34200.00\t34800.00\t35400.00\t36000.00\t36600.00\t37200.00\t37800.00\t38400.00\t39000.00\t39600.00\t40200.00\t40800.00\t41400.00\t42000.00\t42600.00\t43200.00\t43800.00\t44400.00\t45000.00\t45600.00\t46200.00\t46800.00\t47400.00\t48000.00\t48600.00\t49200.00\t49800.00\t50400.00\t51000.00\t51600.00\t52200.00\t52800.00\t53400.00\t54000.00\t54600.00\t55200.00\t55800.00\t56400.00\t57000.00\t57600.00\t58200.00\t58800.00\t59400.00\t60000.00\t60600.00\t61200.00\t61800.00\t62400.00\t63000.00\t63600.00\t64200.00\t64800.00\t65400.00\t66000.00\t66600.00\t67200.00\t67800.00\t68400.00\t69000.00\t69600.00\t70200.00\t70800.00\t71400.00\t72000.00\t72600.00\t73200.00\t73800.00\t74400.00\t75000.00\t75600.00\t76200.00\t76800.00\t77400.00\t78000.00\t78600.00\t79200.00\t79800.00\t80400.00\t81000.00\t81600.00\t82200.00\t82800.00\t83400.00\t84000.00\t84600.00\t85200.00\t85800.00\t86400.00]"  BeginIndexSearchUsingPreviousIndexResult=on  Table="[179.5\t163.3\t152.9\t132.5\t118.9\t111.3\t124.6\t103.3\t83.5\t81.2\t85.9\t85.2\t91.9\t95.6\t95.9\t81.8\t83.7\t86.7\t93.8\t81.2\t92.7\t99.4\t112.6\t88.2\t85.6\t78.4\t88.4\t93.9\t86.1\t86.0\t111.7\t143.5\t122.7\t136.8\t142.2\t135.1\t145.6\t141.8\t152.1\t140.3\t167.9\t256.6\t226.1\t263.8\t283.9\t303.3\t279.5\t294.9\t282.3\t288.8\t333.5\t360.9\t421.4\t494.2\t392.5\t439.7\t395.9\t394.4\t364.9\t353.0\t359.1\t370.9\t398.5\t447.4\t344.5\t330.8\t306.8\t331.3\t331.9\t307.6\t371.3\t387.4\t376.6\t360.2\t414.1\t445.1\t411.1\t389.5\t425.2\t340.0\t316.3\t332.8\t352.3\t301.8\t261.8\t298.1\t350.9\t327.8\t296.5\t319.6\t368.4\t327.2\t265.7\t277.9\t292.9\t301.4\t377.9\t336.0\t324.6\t353.8\t389.7\t355.9\t328.4\t325.9\t378.1\t338.0\t379.1\t414.8\t418.1\t464.8\t488.1\t489.1\t485.7\t581.3\t579.7\t526.2\t551.4\t618.6\t628.5\t578.8\t553.3\t481.5\t455.6\t487.9\t507.3\t497.6\t515.4\t510.2\t490.5\t500.5\t494.1\t532.9\t506.5\t466.6\t438.0\t385.4\t381.2\t385.9\t351.7\t371.3\t340.8\t320.2\t277.0\t228.9\t179.5]"  InternalRulePriority=Speed  RndMeth=Simplest  InputSameDT=on
  Magnitude-Angle to Complex1 : MagnitudeAngleToComplex
  Snubber3 : powerlib/Elements/Series RLC Branch  LConnTagsString=__new0  RConnTagsString=__new0  BranchType=R  Resistance=1e6  Inductance=1e-3  SetiL0=off  InitialCurrent=0  Capacitance=1e-6  Setx0=off  InitialVoltage=0  Measurements=None
      settings: SourceProductName=Simscape Electrical
  meas cur2 : powerlib/Measurements/Current Measurement  PhasorSimulation=on  OutputType=Complex  PSBequivalent=0
      settings: SourceProductName=Simscape Electrical
  Conn1 : PMIOPort  Side=Left
  Conn2 : PMIOPort  Port=2  Side=Right
  Out1 : Outport
  wires:
  Magnitude-Angle to Complex1/1 -> Controlled Current Source4/1
  meas cur2/1 -> Out1/1
  Clock/1 -> Load Data 1-D Lookup Table/1
  Load Data 1-D Lookup Table/1 -> Gain6/1
  [Vsec] -> Complex to Magnitude-Angle/1
  Gain6/1 -> Gain10/1
  Gain10/1 -> Magnitude-Angle to Complex1/1
  Complex to Magnitude-Angle/1 -> Magnitude-Angle to Complex1/2
  connections:
  meas cur2/LConn1 -- Conn1/RConn1
  Snubber3/LConn1 -- Controlled Current Source4/RConn1 -- meas cur2/RConn1
  Snubber3/RConn1 -- Controlled Current Source4/LConn1 -- Conn2/RConn1

== system power_microgrid_v5_battery/House 9 ==
  Clock : Clock
  Complex to Magnitude-Angle : ComplexToMagnitudeAngle  Output=Angle
  Controlled Current Source4 : powerlib/Electrical Sources/Controlled Current Source  Initialize=on  Source_Type=AC  Amplitude=0  Phase=0  Frequency=50  Measurements=None
      settings: SourceProductName=Simscape Electrical
  Gain10 : Gain  Gain=sqrt(2)
  Gain6 : Gain  Gain=-1/230
  Load Data 1-D Lookup Table : Lookup_n-D  NumberOfTableDimensions=1  BreakpointsForDimension1="[0.00\t600.00\t1200.00\t1800.00\t2400.00\t3000.00\t3600.00\t4200.00\t4800.00\t5400.00\t6000.00\t6600.00\t7200.00\t7800.00\t8400.00\t9000.00\t9600.00\t10200.00\t10800.00\t11400.00\t12000.00\t12600.00\t13200.00\t13800.00\t14400.00\t15000.00\t15600.00\t16200.00\t16800.00\t17400.00\t18000.00\t18600.00\t19200.00\t19800.00\t20400.00\t21000.00\t21600.00\t22200.00\t22800.00\t23400.00\t24000.00\t24600.00\t25200.00\t25800.00\t26400.00\t27000.00\t27600.00\t28200.00\t28800.00\t29400.00\t30000.00\t30600.00\t31200.00\t31800.00\t32400.00\t33000.00\t33600.00\t34200.00\t34800.00\t35400.00\t36000.00\t36600.00\t37200.00\t37800.00\t38400.00\t39000.00\t39600.00\t40200.00\t40800.00\t41400.00\t42000.00\t42600.00\t43200.00\t43800.00\t44400.00\t45000.00\t45600.00\t46200.00\t46800.00\t47400.00\t48000.00\t48600.00\t49200.00\t49800.00\t50400.00\t51000.00\t51600.00\t52200.00\t52800.00\t53400.00\t54000.00\t54600.00\t55200.00\t55800.00\t56400.00\t57000.00\t57600.00\t58200.00\t58800.00\t59400.00\t60000.00\t60600.00\t61200.00\t61800.00\t62400.00\t63000.00\t63600.00\t64200.00\t64800.00\t65400.00\t66000.00\t66600.00\t67200.00\t67800.00\t68400.00\t69000.00\t69600.00\t70200.00\t70800.00\t71400.00\t72000.00\t72600.00\t73200.00\t73800.00\t74400.00\t75000.00\t75600.00\t76200.00\t76800.00\t77400.00\t78000.00\t78600.00\t79200.00\t79800.00\t80400.00\t81000.00\t81600.00\t82200.00\t82800.00\t83400.00\t84000.00\t84600.00\t85200.00\t85800.00\t86400.00]"  BeginIndexSearchUsingPreviousIndexResult=on  Table="[179.5\t163.3\t152.9\t132.5\t118.9\t111.3\t124.6\t103.3\t83.5\t81.2\t85.9\t85.2\t91.9\t95.6\t95.9\t81.8\t83.7\t86.7\t93.8\t81.2\t92.7\t99.4\t112.6\t88.2\t85.6\t78.4\t88.4\t93.9\t86.1\t86.0\t111.7\t143.5\t122.7\t136.8\t142.2\t135.1\t145.6\t141.8\t152.1\t140.3\t167.9\t256.6\t226.1\t263.8\t283.9\t303.3\t279.5\t294.9\t282.3\t288.8\t333.5\t360.9\t421.4\t494.2\t392.5\t439.7\t395.9\t394.4\t364.9\t353.0\t359.1\t370.9\t398.5\t447.4\t344.5\t330.8\t306.8\t331.3\t331.9\t307.6\t371.3\t387.4\t376.6\t360.2\t414.1\t445.1\t411.1\t389.5\t425.2\t340.0\t316.3\t332.8\t352.3\t301.8\t261.8\t298.1\t350.9\t327.8\t296.5\t319.6\t368.4\t327.2\t265.7\t277.9\t292.9\t301.4\t377.9\t336.0\t324.6\t353.8\t389.7\t355.9\t328.4\t325.9\t378.1\t338.0\t379.1\t414.8\t418.1\t464.8\t488.1\t489.1\t485.7\t581.3\t579.7\t526.2\t551.4\t618.6\t628.5\t578.8\t553.3\t481.5\t455.6\t487.9\t507.3\t497.6\t515.4\t510.2\t490.5\t500.5\t494.1\t532.9\t506.5\t466.6\t438.0\t385.4\t381.2\t385.9\t351.7\t371.3\t340.8\t320.2\t277.0\t228.9\t179.5]"  InternalRulePriority=Speed  RndMeth=Simplest  InputSameDT=on
  Magnitude-Angle to Complex1 : MagnitudeAngleToComplex
  Snubber3 : powerlib/Elements/Series RLC Branch  LConnTagsString=__new0  RConnTagsString=__new0  BranchType=R  Resistance=1e6  Inductance=1e-3  SetiL0=off  InitialCurrent=0  Capacitance=1e-6  Setx0=off  InitialVoltage=0  Measurements=None
      settings: SourceProductName=Simscape Electrical
  meas cur2 : powerlib/Measurements/Current Measurement  PhasorSimulation=on  OutputType=Complex  PSBequivalent=0
      settings: SourceProductName=Simscape Electrical
  Conn1 : PMIOPort  Side=Left
  Conn2 : PMIOPort  Port=2  Side=Right
  Out1 : Outport
  wires:
  meas cur2/1 -> Out1/1
  Clock/1 -> Load Data 1-D Lookup Table/1
  Magnitude-Angle to Complex1/1 -> Controlled Current Source4/1
  Load Data 1-D Lookup Table/1 -> Gain6/1
  Complex to Magnitude-Angle/1 -> Magnitude-Angle to Complex1/2
  Gain10/1 -> Magnitude-Angle to Complex1/1
  Gain6/1 -> Gain10/1
  [Vsec] -> Complex to Magnitude-Angle/1
  connections:
  Controlled Current Source4/LConn1 -- Conn2/RConn1 -- Snubber3/RConn1
  Controlled Current Source4/RConn1 -- meas cur2/RConn1 -- Snubber3/LConn1
  Conn1/RConn1 -- meas cur2/LConn1

== system power_microgrid_v5_battery/PV ==
  Clock : Clock
  Complex to Magnitude-Angle : ComplexToMagnitudeAngle  Output=Angle
  Controlled Current Source : powerlib/Electrical Sources/Controlled Current Source  Initialize=on  Source_Type=AC  Amplitude=0  Phase=0  Frequency=50  Measurements=None
      settings: SourceProductName=Simscape Electrical
  Gain10 : Gain  Gain=sqrt(2)
  Gain5 : Gain  Gain=1/230
  Ground2 : powerlib/Elements/Ground  LConnTagsString=a
      settings: SourceProductName=Simscape Electrical
  Magnitude-Angle to Complex1 : MagnitudeAngleToComplex
  Snubber1 : powerlib/Elements/Series RLC Branch  LConnTagsString=__new0  RConnTagsString=__new0  BranchType=R  Resistance=1e6  Inductance=1e-3  SetiL0=off  InitialCurrent=0  Capacitance=1e-6  Setx0=off  InitialVoltage=0  Measurements=None
      settings: SourceProductName=Simscape Electrical
  Solar Data 1-D Lookup Table : Lookup_n-D  NumberOfTableDimensions=1  BreakpointsForDimension1=SPT_1min  BeginIndexSearchUsingPreviousIndexResult=on  Table=SPD_1min  InternalRulePriority=Speed  RndMeth=Simplest  InputSameDT=on
  meas cur3 : powerlib/Measurements/Current Measurement  PhasorSimulation=on  OutputType=Complex  PSBequivalent=0
      settings: SourceProductName=Simscape Electrical
  Conn1 : PMIOPort  Side=Left
  Out1 : Outport
  wires:
  meas cur3/1 -> Out1/1
  Magnitude-Angle to Complex1/1 -> Controlled Current Source/1
  Clock/1 -> Solar Data 1-D Lookup Table/1
  Solar Data 1-D Lookup Table/1 -> Gain5/1
  Gain5/1 -> Gain10/1
  Gain10/1 -> Magnitude-Angle to Complex1/1
  Complex to Magnitude-Angle/1 -> Magnitude-Angle to Complex1/2
  [Vsec] -> Complex to Magnitude-Angle/1
  connections:
  Ground2/LConn1 -- Controlled Current Source/LConn1 -- Snubber1/RConn1
  Snubber1/LConn1 -- Controlled Current Source/RConn1 -- meas cur3/LConn1
  Conn1/RConn1 -- meas cur3/RConn1
